simulink model "k1vispr2t"  (Simulink 8.8)
settings: Solver=ode45  StartTime=0.0  StopTime=10.0  RelTol=1e-3  EnableMultiTasking=on
libraries: cdsIPCx x6, cdsEpicsOut x6, cdsBit2Word x6, cdsCDI64 x3, cdsCDO64 x3, cdsEpicsBinIn x3, cdsWord2Bit x3, dac x2, cdsAdcx0 x1, cdsCDO32 x1, TOWER_MASTER x1, BO_TYPEBP_MASTER x1
settings Model: SuppressorTable=22 serialization::archive 11 0 3 0 0 0 11 0  Creator=controls  LastModifiedBy=controls
settings OptimizationCC: ExpressionDepthLimit=2147483647  InitFltsAndDblsToZero=on
settings DebuggingCC: SolverPrmCheckMsg=warning  AllowSymbolicDim=off  StrictBusMsg=Warning

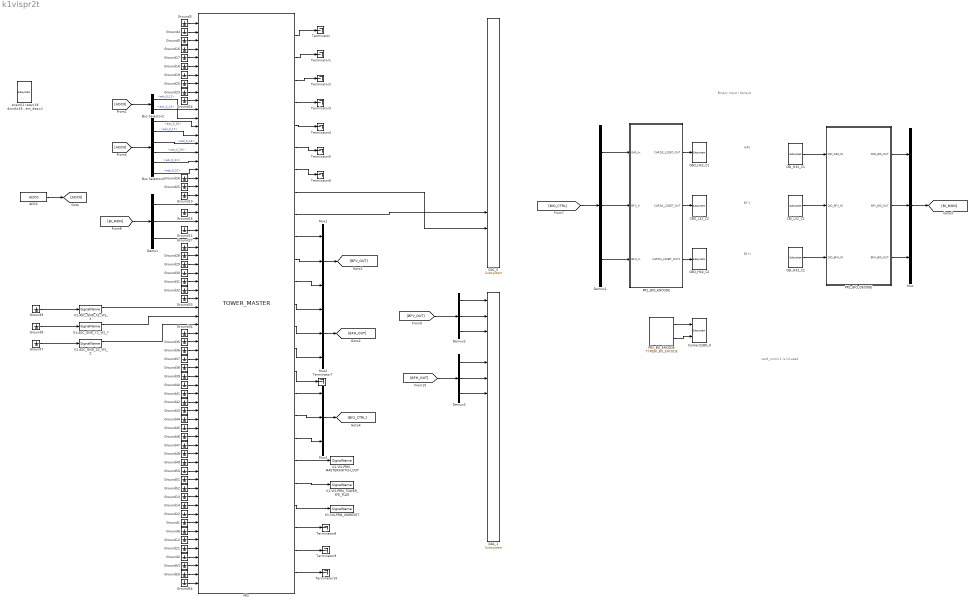
== system k1vispr2t ==
  note: Binary Input / Output
  note: card_num=1 is Unused
  note: GAS
  note: BF V
  note: BF H
  ADC0 : cdsAdcx0/ADC0  Tag=cdsAdc  Description=|
      | type-GSC_16AI64SSA
      | card_num=0
      settings: AttributesFormatString=%<Description>\n%<Tag>
  Bus Selector2 : BusSelector  Description=ADC Selector  OutputSignals=adc_0_12,adc_0_13
      settings: AttributesFormatString=%<Description>
  Bus Selector4 : BusSelector  Description=ADC Selector  OutputSignals=adc_0_16,adc_0_17,adc_0_18,adc_0_20,adc_0_21,adc_0_22
      settings: AttributesFormatString=%<Description>
  CBI_H32_C1 : cdsCDI64/Subsystem  Tag=cdsCDI64  Description=card_num=3
      settings: AttributesFormatString=%<Tag>\n%<Description>
  CBI_H32_C2 : cdsCDI64/Subsystem  Tag=cdsCDI64  Description=card_num=5
      settings: AttributesFormatString=%<Tag>\n%<Description>
  CBI_L32_C2 : cdsCDI64/Subsystem  Tag=cdsCDI64  Description=card_num=4
      settings: AttributesFormatString=%<Tag>\n%<Description>
  CBO_H32_C1 : cdsCDO64/Subsystem  Tag=cdsCDO64  Description=card_num=3
      settings: AttributesFormatString=%<Tag>\n%<Description>
  CBO_H32_C2 : cdsCDO64/Subsystem  Tag=cdsCDO64  Description=card_num=5
      settings: AttributesFormatString=%<Tag>\n%<Description>
  CBO_L32_C2 : cdsCDO64/Subsystem  Tag=cdsCDO64  Description=card_num=4
      settings: AttributesFormatString=%<Tag>\n%<Description>
  Contec32BO_0 : cdsCDO32/Subsystem  Tag=cdsCDO32  Description=Contec32 bit binary output module driver
      settings: AttributesFormatString=%<Tag>
  DAC_0 : dac/Subsystem  Description=|
      | type=GSC_16AO16,
      | card_num=0
      settings: AttributesFormatString=%<Description>
  DAC_1 : dac/Subsystem  Description=|
      | type=GSC_16AO16,
      | card_num=1
      settings: AttributesFormatString=%<Description>
  Demux{,1..3} (4 alike) : Demux  Outputs=3
  Ground{1..55} (55 alike) : Ground
  K1:ASC_GND_X2_VIS_X : cdsIPCx/SignalName  Tag=cdsIPCx_PCIE  Description=Inter-Process Communication via PCI Express network.
      settings: AttributesFormatString=%<Tag>
  K1:ASC_GND_Y2_VIS_Y : cdsIPCx/SignalName  Tag=cdsIPCx_PCIE  Description=Inter-Process Communication via PCI Express network.
      settings: AttributesFormatString=%<Tag>
  K1:ASC_GND_Z2_VIS_Z : cdsIPCx/SignalName  Tag=cdsIPCx_PCIE  Description=Inter-Process Communication via PCI Express network.
      settings: AttributesFormatString=%<Tag>
  K1:VIS-PRM_MASTERSWITCH_OUT : cdsIPCx/SignalName  Tag=cdsIPCx_SHMEM  Description=Inter-Process Communication via Shared memory.
      settings: AttributesFormatString=%<Tag>
  K1:VIS-PRM_TOWER_WD_FLAG : cdsIPCx/SignalName  Tag=cdsIPCx_SHMEM  Description=Inter-Process Communication via Shared memory.
      settings: AttributesFormatString=%<Tag>
  K1:VIS-PRM_WDRESET : cdsIPCx/SignalName  Tag=cdsIPCx_SHMEM  Description=Inter-Process Communication via Shared memory.
      settings: AttributesFormatString=%<Tag>
  Mux{,1..3} (4 alike) : Mux  Inputs=3
  PR2 : TOWER_MASTER/TOWER_MASTER
  PR2_BIO_DECODE : Subsystem
  PR2_BIO_ENCODE : Subsystem
  PR2_BO_ENCODE : BO_TYPEBP_MASTER/TYPEBP_BO_ENCODE
  Terminator{,1..10} (11 alike) : Terminator
  site=K1 rate=2K dcuid=45 host=k1pr2 specific_cpu=2 adcSlave=1 shmem_daq=1 : cdsParameters/Subsystem  Tag=cdsParameters  Description=|
      | Purpose:                                                                                                                                                                                                                                
      | Provide system parameters to the FE code generator to properly configure the generated EPICS names, rep rate of the FE controller, and the Data Acquisition node ID for proper storage of data from this FE controller.                 
      |                                                                                                                                                                                                                                         
      | Useage:                                                                                                                                                                                                                                 
      | The part NAME field is used to identify the FE parameters. It must be of the form:                                                                                                                                                      
      | site=                                                                                                                                                                                                                                   
      | rate=                                                                                                                                                                                                                                   
      | dcuid=                                                                                                                                                                                                                                  
      |                                                                                                                                                                                                                                         
      | Where:                                                                                                                                                                                                                                  
      | site= argument may be H1, H2, L1, M1, G1, either as a single argument or multiple, for example site=H1,H2. These are the only names allowed. These will become the first two characters of all EPICS and signal names (for example G1:).
      |                                                                                                                                                                                                                                         
      | rate= may be 2K, 16K, 32K, or 64K                                                                                                                                                                                                       
      |                                                                                                                                                                                                                                         
      | dcuid= is site specific ie it must be unique at each site.
      settings: AttributesFormatString=%<Tag>
  wires:
  ADC0/1 -> [ADC0]
  [BFV_OUT] -> Demux2/1
  Demux2/1 -> DAC_1/1
  Demux2/2 -> DAC_1/2
  Demux2/3 -> DAC_1/3
  [BFH_OUT] -> Demux3/1
  Demux3/1 -> DAC_1/5
  Demux3/2 -> DAC_1/6
  Demux3/3 -> DAC_1/7
  Bus Selector4/1 -> PR2/13  "<adc_0_16>"
  [ADC0] -> Bus Selector2/1
  Bus Selector4/6 -> PR2/18  "<adc_0_22>"
  [ADC0] -> Bus Selector4/1
  Bus Selector2/1 -> PR2/12  "<adc_0_12>"
  Bus Selector2/2 -> PR2/11  "<adc_0_13>"
  Bus Selector4/2 -> PR2/14  "<adc_0_17>"
  Bus Selector4/3 -> PR2/15  "<adc_0_18>"
  Bus Selector4/4 -> PR2/16  "<adc_0_20>"
  Bus Selector4/5 -> PR2/17  "<adc_0_21>"
  [BI_MON] -> Demux/1
  Demux/1 -> PR2/22
  Demux/2 -> PR2/24
  Demux/3 -> PR2/26
  Ground11/1 -> PR2/25
  Ground15/1 -> PR2/23
  Ground10/1 -> PR2/21
  Mux1/1 -> [BFV_OUT]
  Mux2/1 -> [BFH_OUT]
  Mux3/1 -> [BIO_CTRL]
  PR2_BIO_DECODE/1(GAS_BIO_OUT) -> Mux/1
  Mux/1 -> [BI_MON]
  [BIO_CTRL] -> Demux1/1
  PR2_BIO_ENCODE/2(CARD4_L32BIT_OUT) -> CBO_L32_C2/1
  Demux1/1 -> PR2_BIO_ENCODE/1(GAS_In)
  Demux1/2 -> PR2_BIO_ENCODE/2(BFV_In)
  Demux1/3 -> PR2_BIO_ENCODE/3(BFH_In)
  CBI_H32_C1/1 -> PR2_BIO_DECODE/1(DIO_GAS_IN)
  CBI_L32_C2/1 -> PR2_BIO_DECODE/2(DIO_BFV_IN)
  PR2_BIO_DECODE/2(BFV_BIO_OUT) -> Mux/2
  PR2_BIO_DECODE/3(BFH_BIO_OUT) -> Mux/3
  PR2_BIO_ENCODE/1(CARD3_L32BIT_OUT) -> CBO_H32_C1/1
  PR2_BIO_ENCODE/3(CARD4_L32BIT_OUT1) -> CBO_H32_C2/1
  CBI_H32_C2/1 -> PR2_BIO_DECODE/3(DIO_BFH_IN)
  Ground7/1 -> K1:ASC_GND_Z2_VIS_Z/1
  K1:ASC_GND_Z2_VIS_Z/1 -> PR2/36
  Ground8/1 -> K1:ASC_GND_Y2_VIS_Y/1
  Ground9/1 -> K1:ASC_GND_X2_VIS_X/1
  K1:ASC_GND_X2_VIS_X/1 -> PR2/34
  K1:ASC_GND_Y2_VIS_Y/1 -> PR2/35
  PR2_BO_ENCODE/1 -> Contec32BO_0/1
  PR2_BO_ENCODE/2 -> Contec32BO_0/2
  PR2/9 -> DAC_0/13
  PR2/8 -> DAC_0/14
  PR2/10 -> Mux1/1
  PR2/12 -> Mux1/3
  PR2/11 -> Mux1/2
  PR2/14 -> Mux2/2
  PR2/13 -> Mux2/1
  PR2/15 -> Mux2/3
  PR2/19 -> Mux3/3
  PR2/18 -> Mux3/2
  PR2/17 -> Mux3/1
  Ground21/1 -> PR2/62
  Ground2/1 -> PR2/63
  Ground1/1 -> PR2/59
  Ground6/1 -> PR2/60
  Ground12/1 -> PR2/61
  Ground13/1 -> PR2/56
  Ground14/1 -> PR2/57
  Ground22/1 -> PR2/58
  PR2/20 -> K1:VIS-PRM_MASTERSWITCH_OUT/1
  PR2/22 -> K1:VIS-PRM_WDRESET/1
  PR2/21 -> K1:VIS-PRM_TOWER_WD_FLAG/1
  Ground4/1 -> PR2/2
  Ground3/1 -> PR2/1
  Ground5/1 -> PR2/3
  Ground16/1 -> PR2/4
  Ground17/1 -> PR2/5
  Ground18/1 -> PR2/6
  Ground19/1 -> PR2/7
  Ground20/1 -> PR2/8
  Ground23/1 -> PR2/9
  Ground24/1 -> PR2/10
  Ground25/1 -> PR2/20
  Ground26/1 -> PR2/19
  Ground27/1 -> PR2/27
  Ground28/1 -> PR2/28
  Ground29/1 -> PR2/29
  Ground30/1 -> PR2/30
  Ground31/1 -> PR2/31
  Ground32/1 -> PR2/32
  Ground33/1 -> PR2/33
  Ground34/1 -> PR2/37
  Ground35/1 -> PR2/38
  Ground37/1 -> PR2/40
  Ground36/1 -> PR2/39
  Ground38/1 -> PR2/41
  Ground40/1 -> PR2/43
  Ground39/1 -> PR2/42
  Ground41/1 -> PR2/44
  Ground42/1 -> PR2/45
  Ground43/1 -> PR2/46
  Ground45/1 -> PR2/48
  Ground44/1 -> PR2/47
  Ground46/1 -> PR2/49
  Ground47/1 -> PR2/50
  Ground48/1 -> PR2/51
  Ground49/1 -> PR2/52
  Ground50/1 -> PR2/53
  Ground51/1 -> PR2/54
  Ground52/1 -> PR2/55
  PR2/1 -> Terminator/1
  PR2/2 -> Terminator1/1
  PR2/3 -> Terminator2/1
  PR2/4 -> Terminator3/1
  PR2/5 -> Terminator4/1
  PR2/6 -> Terminator5/1
  PR2/7 -> Terminator6/1
  PR2/16 -> Terminator7/1
  Ground55/1 -> PR2/65
  Ground53/1 -> PR2/64
  Ground54/1 -> PR2/66
  PR2/23 -> Terminator8/1
  PR2/24 -> Terminator9/1
  PR2/25 -> Terminator10/1

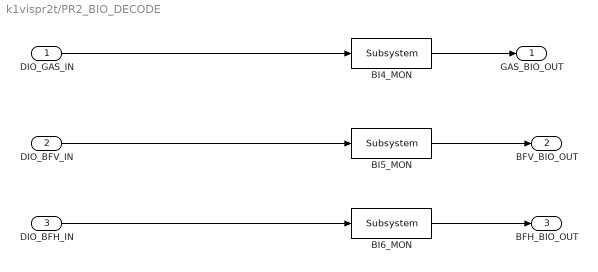
== system k1vispr2t/PR2_BIO_DECODE ==
  DIO_GAS_IN : Inport
  DIO_BFV_IN : Inport  Port=2
  DIO_BFH_IN : Inport  Port=3
  BI4_MON : cdsEpicsOut/Subsystem  Tag=cdsEpicsOutput  Description=|
      | Purpose:                                          
      | Output a FE signal to an EPICS channel.           
      |                                                   
      | Operation:                                        
      | Takes input value and passes it to EPICS record.  
      |                                                   
      | Usage:                                            
      | Name the part with the desired EPICS rrecord name.
      settings: AttributesFormatString=%<Tag>
  BI5_MON : cdsEpicsOut/Subsystem  Tag=cdsEpicsOutput  Description=|
      | Purpose:                                          
      | Output a FE signal to an EPICS channel.           
      |                                                   
      | Operation:                                        
      | Takes input value and passes it to EPICS record.  
      |                                                   
      | Usage:                                            
      | Name the part with the desired EPICS rrecord name.
      settings: AttributesFormatString=%<Tag>
  BI6_MON : cdsEpicsOut/Subsystem  Tag=cdsEpicsOutput  Description=|
      | Purpose:                                          
      | Output a FE signal to an EPICS channel.           
      |                                                   
      | Operation:                                        
      | Takes input value and passes it to EPICS record.  
      |                                                   
      | Usage:                                            
      | Name the part with the desired EPICS rrecord name.
      settings: AttributesFormatString=%<Tag>
  GAS_BIO_OUT : Outport
  BFV_BIO_OUT : Outport  Port=2
  BFH_BIO_OUT : Outport  Port=3
  wires:
  DIO_GAS_IN/1 -> BI4_MON/1
  DIO_BFV_IN/1 -> BI5_MON/1
  BI4_MON/1 -> GAS_BIO_OUT/1
  BI5_MON/1 -> BFV_BIO_OUT/1
  DIO_BFH_IN/1 -> BI6_MON/1
  BI6_MON/1 -> BFH_BIO_OUT/1

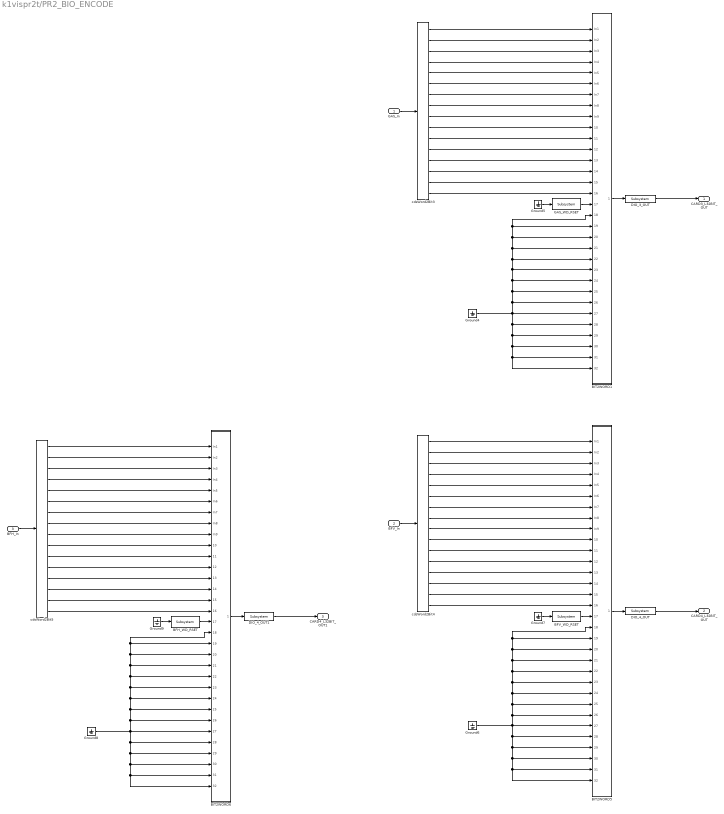
== system k1vispr2t/PR2_BIO_ENCODE ==
  GAS_In : Inport
  BFV_In : Inport  Port=2
  BFH_In : Inport  Port=3
  BFH_WD_RSET : cdsEpicsBinIn/Subsystem  Tag=cdsEpicsBinIn  Description=|
      | Purpose:                                                                            
      | Create an EPICS binary (0 or 1) input channel to the FE realtime controls.          
      |                                                                                     
      | Operation:                                                                          
      | Outputs value from an EPICS ai record. Value is binary input (bi Epics record type).
      |                                                                                     
      | Usage:                                                                              
      | Name the part with the desired EPICS channel name.
      settings: AttributesFormatString=%<Tag>
  BFV_WD_RSET : cdsEpicsBinIn/Subsystem  Tag=cdsEpicsBinIn  Description=|
      | Purpose:                                                                            
      | Create an EPICS binary (0 or 1) input channel to the FE realtime controls.          
      |                                                                                     
      | Operation:                                                                          
      | Outputs value from an EPICS ai record. Value is binary input (bi Epics record type).
      |                                                                                     
      | Usage:                                                                              
      | Name the part with the desired EPICS channel name.
      settings: AttributesFormatString=%<Tag>
  BIT2WORD1 : Subsystem
  BIT2WORD5 : Subsystem
  BIT2WORD6 : Subsystem
  DIO_3_OUT : cdsEpicsOut/Subsystem  Tag=cdsEpicsOutput  Description=|
      | Purpose:                                          
      | Output a FE signal to an EPICS channel.           
      |                                                   
      | Operation:                                        
      | Takes input value and passes it to EPICS record.  
      |                                                   
      | Usage:                                            
      | Name the part with the desired EPICS rrecord name.
      settings: AttributesFormatString=%<Tag>
  DIO_4_OUT : cdsEpicsOut/Subsystem  Tag=cdsEpicsOutput  Description=|
      | Purpose:                                          
      | Output a FE signal to an EPICS channel.           
      |                                                   
      | Operation:                                        
      | Takes input value and passes it to EPICS record.  
      |                                                   
      | Usage:                                            
      | Name the part with the desired EPICS rrecord name.
      settings: AttributesFormatString=%<Tag>
  DIO_4_OUT1 : cdsEpicsOut/Subsystem  Tag=cdsEpicsOutput  Description=|
      | Purpose:                                          
      | Output a FE signal to an EPICS channel.           
      |                                                   
      | Operation:                                        
      | Takes input value and passes it to EPICS record.  
      |                                                   
      | Usage:                                            
      | Name the part with the desired EPICS rrecord name.
      settings: AttributesFormatString=%<Tag>
  GAS_WD_RSET : cdsEpicsBinIn/Subsystem  Tag=cdsEpicsBinIn  Description=|
      | Purpose:                                                                            
      | Create an EPICS binary (0 or 1) input channel to the FE realtime controls.          
      |                                                                                     
      | Operation:                                                                          
      | Outputs value from an EPICS ai record. Value is binary input (bi Epics record type).
      |                                                                                     
      | Usage:                                                                              
      | Name the part with the desired EPICS channel name.
      settings: AttributesFormatString=%<Tag>
  Ground{4..9} (6 alike) : Ground
  cdsWord2Bit3 : cdsWord2Bit/cdsWord2Bit  Tag=cdsWord2Bit  Description=Generate 16 0/1 outputs from single 16-bit integer input
      settings: AttributesFormatString=cdsWord2Bit
  cdsWord2Bit4 : cdsWord2Bit/cdsWord2Bit  Tag=cdsWord2Bit  Description=Generate 16 0/1 outputs from single 16-bit integer input
      settings: AttributesFormatString=cdsWord2Bit
  cdsWord2Bit5 : cdsWord2Bit/cdsWord2Bit  Tag=cdsWord2Bit  Description=Generate 16 0/1 outputs from single 16-bit integer input
      settings: AttributesFormatString=cdsWord2Bit
  CARD3_L32BIT_OUT : Outport
  CARD4_L32BIT_OUT : Outport  Port=2
  CARD4_L32BIT_OUT1 : Outport  Port=3
  wires:
  BIT2WORD1/1(Out1) -> DIO_3_OUT/1
  DIO_3_OUT/1 -> CARD3_L32BIT_OUT/1
  Ground4/1 -> BIT2WORD1/27(In27), BIT2WORD1/26(In26), BIT2WORD1/25(In25), BIT2WORD1/24(In24), BIT2WORD1/23(In23), BIT2WORD1/22(In22), BIT2WORD1/21(In21), BIT2WORD1/20(In20), BIT2WORD1/19(In19), BIT2WORD1/18(In18), BIT2WORD1/28(In28), BIT2WORD1/29(In29), BIT2WORD1/30(In30), BIT2WORD1/32(In32), BIT2WORD1/31(In31)
  GAS_In/1 -> cdsWord2Bit3/1
  cdsWord2Bit3/4 -> BIT2WORD1/4(In4)
  cdsWord2Bit3/5 -> BIT2WORD1/5(In5)
  cdsWord2Bit3/3 -> BIT2WORD1/3(In3)
  cdsWord2Bit3/2 -> BIT2WORD1/2(In2)
  cdsWord2Bit3/6 -> BIT2WORD1/6(In6)
  cdsWord2Bit3/1 -> BIT2WORD1/1(In1)
  cdsWord2Bit3/7 -> BIT2WORD1/7(In7)
  cdsWord2Bit3/8 -> BIT2WORD1/8(In8)
  cdsWord2Bit3/9 -> BIT2WORD1/9(In9)
  cdsWord2Bit3/10 -> BIT2WORD1/10(In10)
  cdsWord2Bit3/11 -> BIT2WORD1/11(In11)
  Ground5/1 -> GAS_WD_RSET/1
  GAS_WD_RSET/1 -> BIT2WORD1/17(In17)
  cdsWord2Bit3/13 -> BIT2WORD1/13(In13)
  cdsWord2Bit3/14 -> BIT2WORD1/14(In14)
  cdsWord2Bit3/15 -> BIT2WORD1/15(In15)
  cdsWord2Bit3/16 -> BIT2WORD1/16(In16)
  cdsWord2Bit3/12 -> BIT2WORD1/12(In12)
  BIT2WORD5/1(Out1) -> DIO_4_OUT/1
  DIO_4_OUT/1 -> CARD4_L32BIT_OUT/1
  Ground6/1 -> BIT2WORD5/27(In27), BIT2WORD5/26(In26), BIT2WORD5/25(In25), BIT2WORD5/24(In24), BIT2WORD5/23(In23), BIT2WORD5/22(In22), BIT2WORD5/21(In21), BIT2WORD5/20(In20), BIT2WORD5/19(In19), BIT2WORD5/18(In18), BIT2WORD5/28(In28), BIT2WORD5/29(In29), BIT2WORD5/30(In30), BIT2WORD5/32(In32), BIT2WORD5/31(In31)
  BFV_In/1 -> cdsWord2Bit4/1
  cdsWord2Bit4/4 -> BIT2WORD5/4(In4)
  cdsWord2Bit4/5 -> BIT2WORD5/5(In5)
  cdsWord2Bit4/3 -> BIT2WORD5/3(In3)
  cdsWord2Bit4/2 -> BIT2WORD5/2(In2)
  cdsWord2Bit4/6 -> BIT2WORD5/6(In6)
  cdsWord2Bit4/1 -> BIT2WORD5/1(In1)
  cdsWord2Bit4/7 -> BIT2WORD5/7(In7)
  cdsWord2Bit4/8 -> BIT2WORD5/8(In8)
  cdsWord2Bit4/9 -> BIT2WORD5/9(In9)
  cdsWord2Bit4/10 -> BIT2WORD5/10(In10)
  cdsWord2Bit4/11 -> BIT2WORD5/11(In11)
  Ground7/1 -> BFV_WD_RSET/1
  BFV_WD_RSET/1 -> BIT2WORD5/17(In17)
  cdsWord2Bit4/13 -> BIT2WORD5/13(In13)
  cdsWord2Bit4/14 -> BIT2WORD5/14(In14)
  cdsWord2Bit4/15 -> BIT2WORD5/15(In15)
  cdsWord2Bit4/16 -> BIT2WORD5/16(In16)
  cdsWord2Bit4/12 -> BIT2WORD5/12(In12)
  BIT2WORD6/1(Out1) -> DIO_4_OUT1/1
  DIO_4_OUT1/1 -> CARD4_L32BIT_OUT1/1
  Ground8/1 -> BIT2WORD6/27(In27), BIT2WORD6/26(In26), BIT2WORD6/25(In25), BIT2WORD6/24(In24), BIT2WORD6/23(In23), BIT2WORD6/22(In22), BIT2WORD6/21(In21), BIT2WORD6/20(In20), BIT2WORD6/19(In19), BIT2WORD6/18(In18), BIT2WORD6/28(In28), BIT2WORD6/29(In29), BIT2WORD6/30(In30), BIT2WORD6/32(In32), BIT2WORD6/31(In31)
  BFH_In/1 -> cdsWord2Bit5/1
  cdsWord2Bit5/4 -> BIT2WORD6/4(In4)
  cdsWord2Bit5/5 -> BIT2WORD6/5(In5)
  cdsWord2Bit5/3 -> BIT2WORD6/3(In3)
  cdsWord2Bit5/2 -> BIT2WORD6/2(In2)
  cdsWord2Bit5/6 -> BIT2WORD6/6(In6)
  cdsWord2Bit5/1 -> BIT2WORD6/1(In1)
  cdsWord2Bit5/7 -> BIT2WORD6/7(In7)
  cdsWord2Bit5/8 -> BIT2WORD6/8(In8)
  cdsWord2Bit5/9 -> BIT2WORD6/9(In9)
  cdsWord2Bit5/10 -> BIT2WORD6/10(In10)
  cdsWord2Bit5/11 -> BIT2WORD6/11(In11)
  Ground9/1 -> BFH_WD_RSET/1
  BFH_WD_RSET/1 -> BIT2WORD6/17(In17)
  cdsWord2Bit5/13 -> BIT2WORD6/13(In13)
  cdsWord2Bit5/14 -> BIT2WORD6/14(In14)
  cdsWord2Bit5/15 -> BIT2WORD6/15(In15)
  cdsWord2Bit5/16 -> BIT2WORD6/16(In16)
  cdsWord2Bit5/12 -> BIT2WORD6/12(In12)

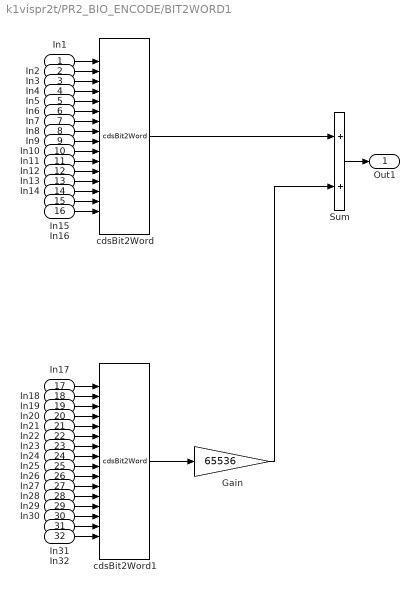
== system k1vispr2t/PR2_BIO_ENCODE/BIT2WORD1 ==
  In1 : Inport
  In2 : Inport  Port=2
  In3 : Inport  Port=3
  In4 : Inport  Port=4
  In5 : Inport  Port=5
  In6 : Inport  Port=6
  In7 : Inport  Port=7
  In8 : Inport  Port=8
  In9 : Inport  Port=9
  In10 : Inport  Port=10
  In11 : Inport  Port=11
  In12 : Inport  Port=12
  In13 : Inport  Port=13
  In14 : Inport  Port=14
  In15 : Inport  Port=15
  In16 : Inport  Port=16
  In17 : Inport  Port=17
  In18 : Inport  Port=18
  In19 : Inport  Port=19
  In20 : Inport  Port=20
  In21 : Inport  Port=21
  In22 : Inport  Port=22
  In23 : Inport  Port=23
  In24 : Inport  Port=24
  In25 : Inport  Port=25
  In26 : Inport  Port=26
  In27 : Inport  Port=27
  In28 : Inport  Port=28
  In29 : Inport  Port=29
  In30 : Inport  Port=30
  In31 : Inport  Port=31
  In32 : Inport  Port=32
  Gain : Gain  Gain=65536
  Sum : Sum
  cdsBit2Word : cdsBit2Word/cdsBit2Word  Tag=cdsBit2Word  Description=Forms single 16 bit integer from 16 0/1 inputs.
      settings: AttributesFormatString=%<Tag>
  cdsBit2Word1 : cdsBit2Word/cdsBit2Word  Tag=cdsBit2Word  Description=Forms single 16 bit integer from 16 0/1 inputs.
      settings: AttributesFormatString=%<Tag>
  Out1 : Outport
  wires:
  Gain/1 -> Sum/2
  cdsBit2Word1/1 -> Gain/1
  cdsBit2Word/1 -> Sum/1
  In1/1 -> cdsBit2Word/1
  In2/1 -> cdsBit2Word/2
  In3/1 -> cdsBit2Word/3
  In4/1 -> cdsBit2Word/4
  In5/1 -> cdsBit2Word/5
  In6/1 -> cdsBit2Word/6
  In7/1 -> cdsBit2Word/7
  In8/1 -> cdsBit2Word/8
  In9/1 -> cdsBit2Word/9
  In10/1 -> cdsBit2Word/10
  Sum/1 -> Out1/1
  In11/1 -> cdsBit2Word/11
  In12/1 -> cdsBit2Word/12
  In13/1 -> cdsBit2Word/13
  In14/1 -> cdsBit2Word/14
  In15/1 -> cdsBit2Word/15
  In16/1 -> cdsBit2Word/16
  In17/1 -> cdsBit2Word1/1
  In18/1 -> cdsBit2Word1/2
  In19/1 -> cdsBit2Word1/3
  In20/1 -> cdsBit2Word1/4
  In21/1 -> cdsBit2Word1/5
  In22/1 -> cdsBit2Word1/6
  In23/1 -> cdsBit2Word1/7
  In24/1 -> cdsBit2Word1/8
  In25/1 -> cdsBit2Word1/9
  In26/1 -> cdsBit2Word1/10
  In27/1 -> cdsBit2Word1/11
  In28/1 -> cdsBit2Word1/12
  In29/1 -> cdsBit2Word1/13
  In30/1 -> cdsBit2Word1/14
  In31/1 -> cdsBit2Word1/15
  In32/1 -> cdsBit2Word1/16

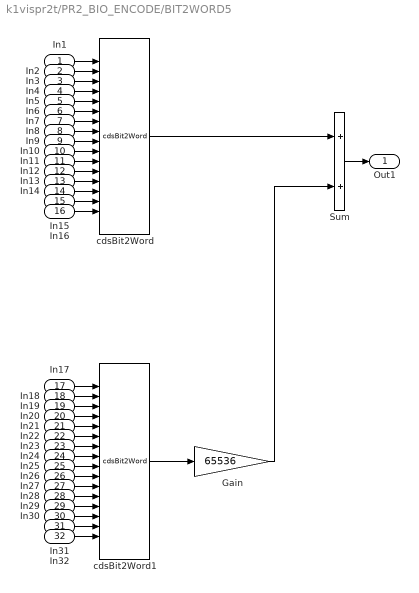
== system k1vispr2t/PR2_BIO_ENCODE/BIT2WORD5 ==
  In1 : Inport
  In2 : Inport  Port=2
  In3 : Inport  Port=3
  In4 : Inport  Port=4
  In5 : Inport  Port=5
  In6 : Inport  Port=6
  In7 : Inport  Port=7
  In8 : Inport  Port=8
  In9 : Inport  Port=9
  In10 : Inport  Port=10
  In11 : Inport  Port=11
  In12 : Inport  Port=12
  In13 : Inport  Port=13
  In14 : Inport  Port=14
  In15 : Inport  Port=15
  In16 : Inport  Port=16
  In17 : Inport  Port=17
  In18 : Inport  Port=18
  In19 : Inport  Port=19
  In20 : Inport  Port=20
  In21 : Inport  Port=21
  In22 : Inport  Port=22
  In23 : Inport  Port=23
  In24 : Inport  Port=24
  In25 : Inport  Port=25
  In26 : Inport  Port=26
  In27 : Inport  Port=27
  In28 : Inport  Port=28
  In29 : Inport  Port=29
  In30 : Inport  Port=30
  In31 : Inport  Port=31
  In32 : Inport  Port=32
  Gain : Gain  Gain=65536
  Sum : Sum
  cdsBit2Word : cdsBit2Word/cdsBit2Word  Tag=cdsBit2Word  Description=Forms single 16 bit integer from 16 0/1 inputs.
      settings: AttributesFormatString=%<Tag>
  cdsBit2Word1 : cdsBit2Word/cdsBit2Word  Tag=cdsBit2Word  Description=Forms single 16 bit integer from 16 0/1 inputs.
      settings: AttributesFormatString=%<Tag>
  Out1 : Outport
  wires:
  Gain/1 -> Sum/2
  cdsBit2Word1/1 -> Gain/1
  cdsBit2Word/1 -> Sum/1
  In1/1 -> cdsBit2Word/1
  In2/1 -> cdsBit2Word/2
  In3/1 -> cdsBit2Word/3
  In4/1 -> cdsBit2Word/4
  In5/1 -> cdsBit2Word/5
  In6/1 -> cdsBit2Word/6
  In7/1 -> cdsBit2Word/7
  In8/1 -> cdsBit2Word/8
  In9/1 -> cdsBit2Word/9
  In10/1 -> cdsBit2Word/10
  Sum/1 -> Out1/1
  In11/1 -> cdsBit2Word/11
  In12/1 -> cdsBit2Word/12
  In13/1 -> cdsBit2Word/13
  In14/1 -> cdsBit2Word/14
  In15/1 -> cdsBit2Word/15
  In16/1 -> cdsBit2Word/16
  In17/1 -> cdsBit2Word1/1
  In18/1 -> cdsBit2Word1/2
  In19/1 -> cdsBit2Word1/3
  In20/1 -> cdsBit2Word1/4
  In21/1 -> cdsBit2Word1/5
  In22/1 -> cdsBit2Word1/6
  In23/1 -> cdsBit2Word1/7
  In24/1 -> cdsBit2Word1/8
  In25/1 -> cdsBit2Word1/9
  In26/1 -> cdsBit2Word1/10
  In27/1 -> cdsBit2Word1/11
  In28/1 -> cdsBit2Word1/12
  In29/1 -> cdsBit2Word1/13
  In30/1 -> cdsBit2Word1/14
  In31/1 -> cdsBit2Word1/15
  In32/1 -> cdsBit2Word1/16

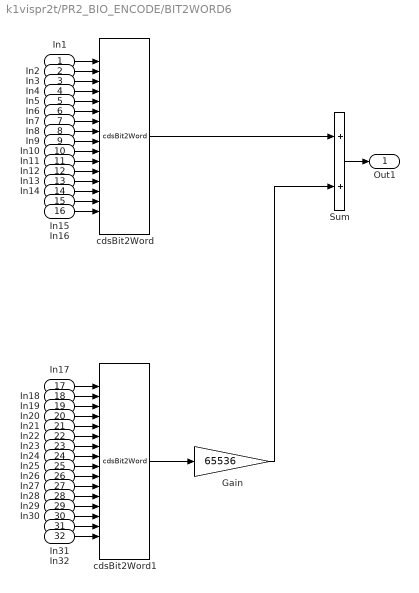
== system k1vispr2t/PR2_BIO_ENCODE/BIT2WORD6 ==
  In1 : Inport
  In2 : Inport  Port=2
  In3 : Inport  Port=3
  In4 : Inport  Port=4
  In5 : Inport  Port=5
  In6 : Inport  Port=6
  In7 : Inport  Port=7
  In8 : Inport  Port=8
  In9 : Inport  Port=9
  In10 : Inport  Port=10
  In11 : Inport  Port=11
  In12 : Inport  Port=12
  In13 : Inport  Port=13
  In14 : Inport  Port=14
  In15 : Inport  Port=15
  In16 : Inport  Port=16
  In17 : Inport  Port=17
  In18 : Inport  Port=18
  In19 : Inport  Port=19
  In20 : Inport  Port=20
  In21 : Inport  Port=21
  In22 : Inport  Port=22
  In23 : Inport  Port=23
  In24 : Inport  Port=24
  In25 : Inport  Port=25
  In26 : Inport  Port=26
  In27 : Inport  Port=27
  In28 : Inport  Port=28
  In29 : Inport  Port=29
  In30 : Inport  Port=30
  In31 : Inport  Port=31
  In32 : Inport  Port=32
  Gain : Gain  Gain=65536
  Sum : Sum
  cdsBit2Word : cdsBit2Word/cdsBit2Word  Tag=cdsBit2Word  Description=Forms single 16 bit integer from 16 0/1 inputs.
      settings: AttributesFormatString=%<Tag>
  cdsBit2Word1 : cdsBit2Word/cdsBit2Word  Tag=cdsBit2Word  Description=Forms single 16 bit integer from 16 0/1 inputs.
      settings: AttributesFormatString=%<Tag>
  Out1 : Outport
  wires:
  Gain/1 -> Sum/2
  cdsBit2Word1/1 -> Gain/1
  cdsBit2Word/1 -> Sum/1
  In1/1 -> cdsBit2Word/1
  In2/1 -> cdsBit2Word/2
  In3/1 -> cdsBit2Word/3
  In4/1 -> cdsBit2Word/4
  In5/1 -> cdsBit2Word/5
  In6/1 -> cdsBit2Word/6
  In7/1 -> cdsBit2Word/7
  In8/1 -> cdsBit2Word/8
  In9/1 -> cdsBit2Word/9
  In10/1 -> cdsBit2Word/10
  Sum/1 -> Out1/1
  In11/1 -> cdsBit2Word/11
  In12/1 -> cdsBit2Word/12
  In13/1 -> cdsBit2Word/13
  In14/1 -> cdsBit2Word/14
  In15/1 -> cdsBit2Word/15
  In16/1 -> cdsBit2Word/16
  In17/1 -> cdsBit2Word1/1
  In18/1 -> cdsBit2Word1/2
  In19/1 -> cdsBit2Word1/3
  In20/1 -> cdsBit2Word1/4
  In21/1 -> cdsBit2Word1/5
  In22/1 -> cdsBit2Word1/6
  In23/1 -> cdsBit2Word1/7
  In24/1 -> cdsBit2Word1/8
  In25/1 -> cdsBit2Word1/9
  In26/1 -> cdsBit2Word1/10
  In27/1 -> cdsBit2Word1/11
  In28/1 -> cdsBit2Word1/12
  In29/1 -> cdsBit2Word1/13
  In30/1 -> cdsBit2Word1/14
  In31/1 -> cdsBit2Word1/15
  In32/1 -> cdsBit2Word1/16
